simulink model "she"  (Simulink 8.1)
settings: Solver=ode45  StartTime=0.0  StopTime=0.2  RelTol=1e-3
InitFcn:
  | % -------------------------------------------------------------------------
  | %  NEWTON-RAPHSON
  | %    Selective Harmonic Elimination (3,5,7,9)
  | %  ------------------------------------------------------------------------
  | 
  | 
  | clc;
  | clear all;
  | 
  | 
  | m1=0:0.01:1;               % Modulation Index
  | 
  | 
  | for ii=1:101               %
  | a1=20*pi/180;          % Initial angles
  | a2=30*pi/180;
  | a3=50*pi/180;
  | a4=70*pi/180;
  | a5=80*pi/180;
  | 
  | 
  | 
  | for i=1:100                %
  | 
  | 
  | T=[m1(ii)*pi/4 0 0 0 0]';
  | 
  | F=[cos(a1)-cos(a2)+cos(a3)-cos(a4)+cos(a5);
  |     cos(3*a1)-cos(3*a2)+cos(3*a3)-cos(3*a4)+cos(3*a5);
  |     cos(5*a1)-cos(5*a2)+cos(5*a3)-cos(5*a4)+cos(5*a5);
  |     cos(7*a1)-cos(7*a2)+cos(7*a3)-cos(7*a4)+cos(7*a5);
  |     cos(9*a1)-cos(9*a2)+cos(9*a3)-cos(9*a4)+cos(9*a5)];
  | 
  | dF=[-sin(a1) +sin(a2) -sin(a3) +sin(a4) -sin(a5);
  |     -3*sin(3*a1) +3*sin(3*a2) -3*sin(3*a3) +3*sin(3*a4) -3*sin(3*a5);
  |     -5*sin(5*a1) +5*sin(5*a2) -5*sin(5*a3) +5*sin(5*a4) -5*sin(5*a5);
  |     -7*sin(7*a1) +7*sin(7*a2) -7*sin(7*a3) +7*sin(7*a4) -7*sin(7*a5);
  |     -9*sin(9*a1) +9*sin(9*a2) -9*sin(9*a3) +9*sin(9*a4) -9*sin(9*a5)];
  | 
  | 
  | % -------------------------------------------------------------------------
  | %                                   Solution
  | % -------------------------------------------------------------------------
  | 
  | 
  | deriv_a=(inv(dF))*(T-F);
  | 
  | alpha=[a1;a2;a3;a4;a5]*180/pi;
  | 
  | deriv_a*180/pi;
  | a1=a1+deriv_a(1);
  | a2=a2+deriv_a(2);
  | a3=a3+deriv_a(3);
  | a4=a4+deriv_a(4);
  | a5=a5+deriv_a(5);
  | if deriv_a>-1e-15 & deriv_a<1e-15
  |     break;
  | end
  | end
  | 
  | a11(ii)=a1*180/pi;
  | a22(ii)=a2*180/pi;
  | a33(ii)=a3*180/pi;
  | a44(ii)=a4*180/pi;
  | a55(ii)=a5*180/pi;
  | end
  | plot(m1,a11,'b',m1,a22,'r',m1,a33,'g',m1,a44,'k',m1,a55,'m');
  | legend('alpha1','alpha2','alpha3','alpha4','alpha5')
  | grid on;
  | title ('Selective Harmonic Elimination - Angles Vs Modulation Index')
  | xlabel('Modulation Index (m)');
  | ylabel('Angles (deg)');
  | 
  | 
  | clc
  | % To choose  the modulation Index---> do ii = (m)*10 - 1
  | ii = 91; % m = 0.9;
  | 
  | a1 = a11(ii);
  | a2 = a22(ii);
  | a3 = a33(ii);
  | a4 = a44(ii);
  | a5= a55(ii);
  | 
  | ang = [ a1 a2 a3 a4 a5]'
libraries: powerlib x9
settings Model: Creator=abdul haleem shaik  LastModifiedBy=Alves
settings DebuggingCC: StrictBusMsg=Warning

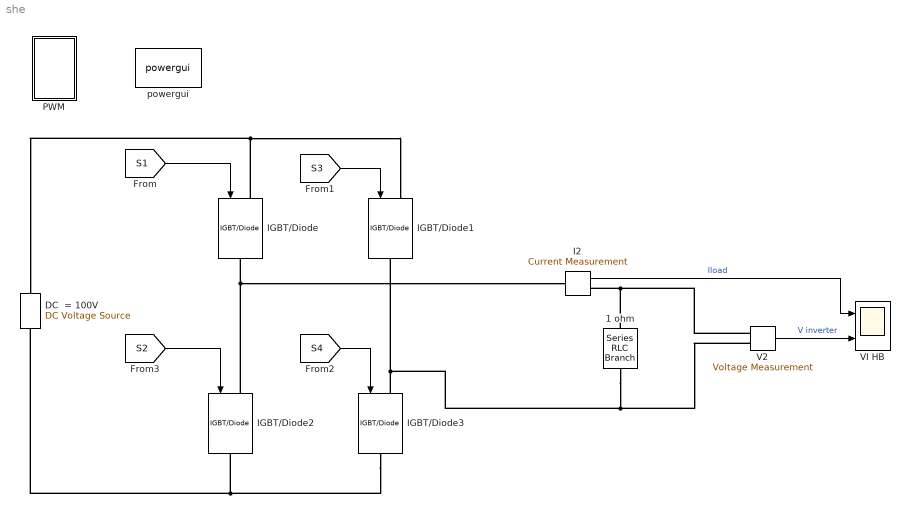
== system she ==
  "1 ohm " : powerlib/Elements/Series RLC Branch  LConnTagsString=__new0  RConnTagsString=__new0  BranchType=R  Resistance=1  Inductance=100e-03  SetiL0=off  InitialCurrent=0  Capacitance=1.0  Setx0=off  InitialVoltage=0  Measurements=None
  DC  = 100V : powerlib/Electrical Sources/DC Voltage Source  Amplitude=100  Measurements=None
  I2 : powerlib/Measurements/Current Measurement  Tag=PoWeRsYsTeMmEaSuReMeNt  PhasorSimulation=off  OutputType=Magnitude  PSBequivalent=0
  IGBT/Diode{,1..3} (4 alike) : powerlib/Power Electronics/IGBT//Diode  Ron=1e-3  Rs=1e5  Cs=inf  Measurements=off
  PWM : Subsystem
  V2 : powerlib/Measurements/Voltage Measurement  Tag=PoWeRsYsTeMmEaSuReMeNt  PhasorSimulation=off  OutputType=Magnitude  PSBequivalent=0
  VI HB : Scope  NumInputPorts=2
      settings: TimeRange=0.1  YMin=-100~-300  YMax=100~300  SaveName=HB  MaxDataPoints=500000
  powergui : powerlib/powergui  Priority=1  SimulationMode=Discrete  SolverType=Tustin  SampleTime=1e-6  frequency=60  SPID=off  DisableSnubberDevices=off  DisableRonSwitches=off  DisableVfSwitches=off  SwTol=0  Interpol=off  DisplayEquations=off  frequencyindice=0  Pbase=100e6  ErrMax=1e-4  Iterations=50  UnitsV=kV  UnitsW=MW  FunctionMessages=off  echomessages=off  HookPort=off  EnableUseOfTLC=off  x0status=blocks  RestoreLinks=warning  ResistiveCurrentMeasurement=off  Frange=[0:2:500]  Ylog=off  Xlog=on  ShowGrid=off  save=off  variable=ZData  structure=HB  ZoomFFT=off  StartTime=0.0  cycles=1  DisplayStyle=1  fundamental=50  FreqAxis=on  MaxFrequency=1000  frequencyindicesteady=1  RmsSteady=1  display=off  Ts=0  methode=off
  wires:
  [S1] -> IGBT/Diode/1
  [S3] -> IGBT/Diode1/1
  [S4] -> IGBT/Diode3/1
  [S2] -> IGBT/Diode2/1
  V2/1 -> VI HB/2  "V inverter"
  I2/1 -> VI HB/1  "Iload"
  connections:
  IGBT/Diode3/LConn1 -- IGBT/Diode1/RConn1 -- "1 ohm "/RConn1 -- V2/LConn2
  IGBT/Diode/LConn1 -- DC  = 100V/RConn1 -- IGBT/Diode1/LConn1
  IGBT/Diode3/RConn1 -- IGBT/Diode2/RConn1 -- DC  = 100V/LConn1
  IGBT/Diode2/LConn1 -- I2/LConn1 -- IGBT/Diode/RConn1
  "1 ohm "/LConn1 -- V2/LConn1 -- I2/RConn1

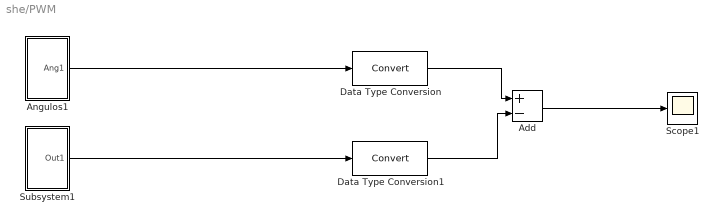
== system she/PWM ==
  Add : Sum  Inputs=+-
  Angulos1 : Subsystem
  Data Type Conversion : DataTypeConversion
  Data Type Conversion1 : DataTypeConversion
  Scope1 : Scope
      settings: SaveName=Pulse
  Subsystem1 : Subsystem
  wires:
  Add/1 -> Scope1/1
  Data Type Conversion/1 -> Add/1
  Data Type Conversion1/1 -> Add/2
  Angulos1/1(Ang1) -> Data Type Conversion/1
  Subsystem1/1(Out1) -> Data Type Conversion1/1

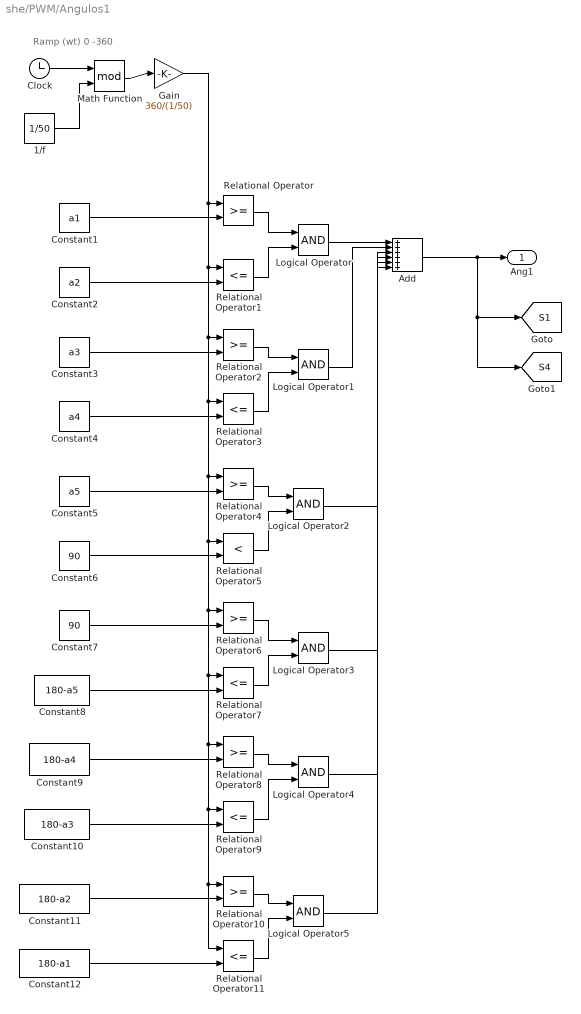
== system she/PWM/Angulos1 ==
  note: Ramp (wt) 0 -360
  1/f : Constant  Value=1/50
  Add : Sum  Inputs=++++++
  Clock : Clock
  Constant1 : Constant  Value=a1
  Constant10 : Constant  Value=180-a3
  Constant11 : Constant  Value=180-a2
  Constant12 : Constant  Value=180-a1
  Constant2 : Constant  Value=a2
  Constant3 : Constant  Value=a3
  Constant4 : Constant  Value=a4
  Constant5 : Constant  Value=a5
  Constant6 : Constant  Value=90
  Constant7 : Constant  Value=90
  Constant8 : Constant  Value=180-a5
  Constant9 : Constant  Value=180-a4
  Gain : Gain  Gain=360/(1/50)
  Logical Operator{,1..5} (6 alike) : Logic  AllPortsSameDT=off  OutDataTypeStr=boolean
  Math Function : Math  Operator=mod  SampleTime=1e-6  SaturateOnIntegerOverflow=on
  Relational Operator{,2,4,6,8,10} (6 alike) : RelationalOperator  OutDataTypeStr=boolean
  Relational Operator{1,3,7,9,11} (5 alike) : RelationalOperator  Operator=<=  OutDataTypeStr=boolean
  Relational Operator5 : RelationalOperator  Operator=<  OutDataTypeStr=boolean
  Ang1 : Outport
  tag scope: S1=global, S4=global
  wires:
  Clock/1 -> Math Function/1
  1/f/1 -> Math Function/2
  Math Function/1 -> Gain/1
  Gain/1 -> Relational Operator/1, Relational Operator1/1, Relational Operator4/1, Relational Operator5/1, Relational Operator8/1, Relational Operator9/1, Relational Operator11/1, Relational Operator10/1, Relational Operator7/1, Relational Operator6/1, Relational Operator3/1, Relational Operator2/1
  Constant1/1 -> Relational Operator/2
  Constant2/1 -> Relational Operator1/2
  Constant3/1 -> Relational Operator2/2
  Constant4/1 -> Relational Operator3/2
  Constant5/1 -> Relational Operator4/2
  Constant6/1 -> Relational Operator5/2
  Relational Operator/1 -> Logical Operator/1
  Relational Operator1/1 -> Logical Operator/2
  Relational Operator2/1 -> Logical Operator1/1
  Relational Operator3/1 -> Logical Operator1/2
  Relational Operator4/1 -> Logical Operator2/1
  Relational Operator5/1 -> Logical Operator2/2
  Logical Operator/1 -> Add/1
  Logical Operator1/1 -> Add/2
  Logical Operator2/1 -> Add/3
  Constant7/1 -> Relational Operator6/2
  Constant8/1 -> Relational Operator7/2
  Constant9/1 -> Relational Operator8/2
  Constant10/1 -> Relational Operator9/2
  Constant11/1 -> Relational Operator10/2
  Constant12/1 -> Relational Operator11/2
  Relational Operator6/1 -> Logical Operator3/1
  Relational Operator7/1 -> Logical Operator3/2
  Relational Operator8/1 -> Logical Operator4/1
  Relational Operator9/1 -> Logical Operator4/2
  Relational Operator10/1 -> Logical Operator5/1
  Relational Operator11/1 -> Logical Operator5/2
  Logical Operator3/1 -> Add/4
  Logical Operator4/1 -> Add/5
  Logical Operator5/1 -> Add/6
  Add/1 -> Ang1/1, [S1], [S4]

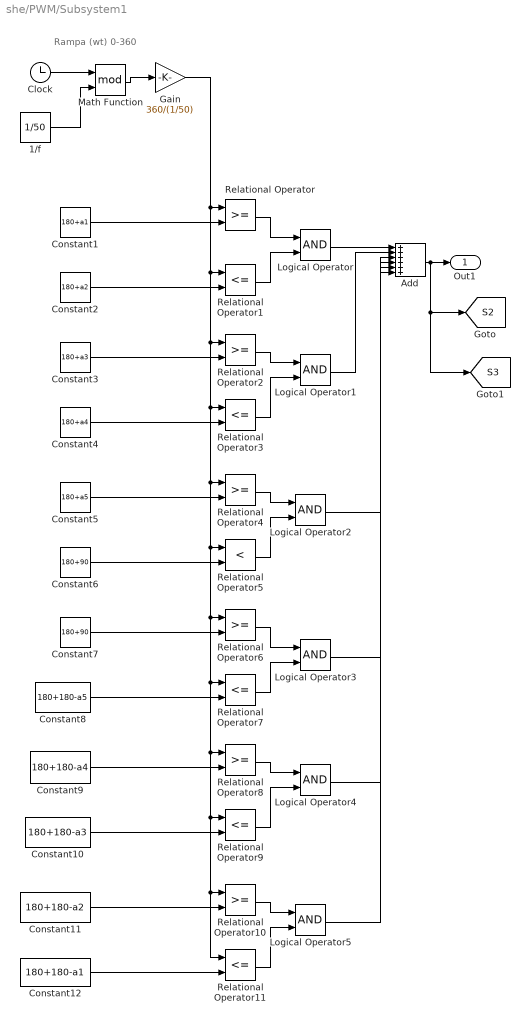
== system she/PWM/Subsystem1 ==
  note: Rampa (wt) 0-360
  1/f : Constant  Value=1/50
  Add : Sum  Inputs=++++++
  Clock : Clock
  Constant1 : Constant  Value=180+a1
  Constant10 : Constant  Value=180+180-a3
  Constant11 : Constant  Value=180+180-a2
  Constant12 : Constant  Value=180+180-a1
  Constant2 : Constant  Value=180+a2
  Constant3 : Constant  Value=180+a3
  Constant4 : Constant  Value=180+a4
  Constant5 : Constant  Value=180+a5
  Constant6 : Constant  Value=180+90
  Constant7 : Constant  Value=180+90
  Constant8 : Constant  Value=180+180-a5
  Constant9 : Constant  Value=180+180-a4
  Gain : Gain  Gain=360/(1/50)
  Logical Operator{,1..5} (6 alike) : Logic  AllPortsSameDT=off  OutDataTypeStr=boolean
  Math Function : Math  Operator=mod  SampleTime=1e-6  SaturateOnIntegerOverflow=on
  Relational Operator{,2,4,6,8,10} (6 alike) : RelationalOperator  OutDataTypeStr=boolean
  Relational Operator{1,3,7,9,11} (5 alike) : RelationalOperator  Operator=<=  OutDataTypeStr=boolean
  Relational Operator5 : RelationalOperator  Operator=<  OutDataTypeStr=boolean
  Out1 : Outport
  tag scope: S2=global, S3=global
  wires:
  Add/1 -> Out1/1, [S2], [S3]
  Logical Operator5/1 -> Add/6
  Logical Operator4/1 -> Add/5
  Logical Operator3/1 -> Add/4
  Relational Operator11/1 -> Logical Operator5/2
  Relational Operator10/1 -> Logical Operator5/1
  Relational Operator9/1 -> Logical Operator4/2
  Relational Operator8/1 -> Logical Operator4/1
  Relational Operator7/1 -> Logical Operator3/2
  Relational Operator6/1 -> Logical Operator3/1
  Constant12/1 -> Relational Operator11/2
  Constant11/1 -> Relational Operator10/2
  Constant10/1 -> Relational Operator9/2
  Constant9/1 -> Relational Operator8/2
  Constant8/1 -> Relational Operator7/2
  Constant7/1 -> Relational Operator6/2
  Logical Operator2/1 -> Add/3
  Logical Operator1/1 -> Add/2
  Logical Operator/1 -> Add/1
  Relational Operator5/1 -> Logical Operator2/2
  Relational Operator4/1 -> Logical Operator2/1
  Relational Operator3/1 -> Logical Operator1/2
  Relational Operator2/1 -> Logical Operator1/1
  Relational Operator1/1 -> Logical Operator/2
  Relational Operator/1 -> Logical Operator/1
  Constant6/1 -> Relational Operator5/2
  Constant5/1 -> Relational Operator4/2
  Constant4/1 -> Relational Operator3/2
  Constant3/1 -> Relational Operator2/2
  Constant2/1 -> Relational Operator1/2
  Constant1/1 -> Relational Operator/2
  Gain/1 -> Relational Operator2/1, Relational Operator3/1, Relational Operator6/1, Relational Operator7/1, Relational Operator10/1, Relational Operator11/1, Relational Operator9/1, Relational Operator8/1, Relational Operator5/1, Relational Operator4/1, Relational Operator1/1, Relational Operator/1
  Math Function/1 -> Gain/1
  1/f/1 -> Math Function/2
  Clock/1 -> Math Function/1
